simulink model "CardiacDigitalTwin_v2"  (R2026a)
settings: Solver=ode45  StopTime=3600  MaxStep=10
values from neighbouring files (symbols this model uses):
  baroreflex_gain = 0.30    (= 0.3)    [cardiac_params_v2.m]
  baroreflex_tau = 60    [cardiac_params_v2.m]
  baseline_heart_rate = 75    [cardiac_params.m]
  beta_blocker_dose_mg = 60    [cardiac_params.m]
  ec50_mg = 35    [cardiac_params_v2.m]
  emax_bpm = 18    [cardiac_params_v2.m]
  hill_n = 1.5    [cardiac_params_v2.m]
  map_setpoint_mmHg = 94    [cardiac_params_v2.m]
  pk_time_constant = 1800    [cardiac_params.m]
  stroke_volume_mL = 70    [cardiac_params.m]
  svr_mmHg_min_per_L = 18    [cardiac_params.m]
settings Model: Creator=tauilsamuel  LastModifiedBy=tauilsamuel

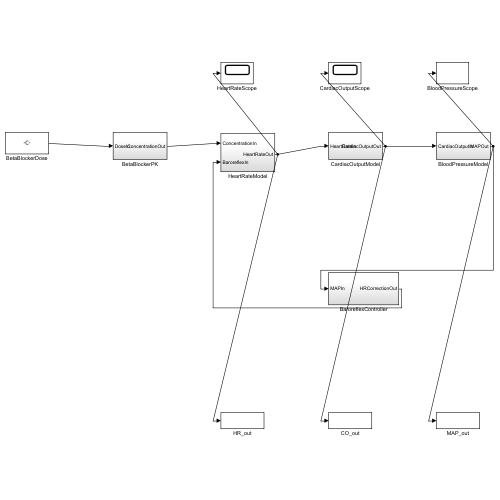
[thumbnail: Simulink's stored preview of the top-level diagram]
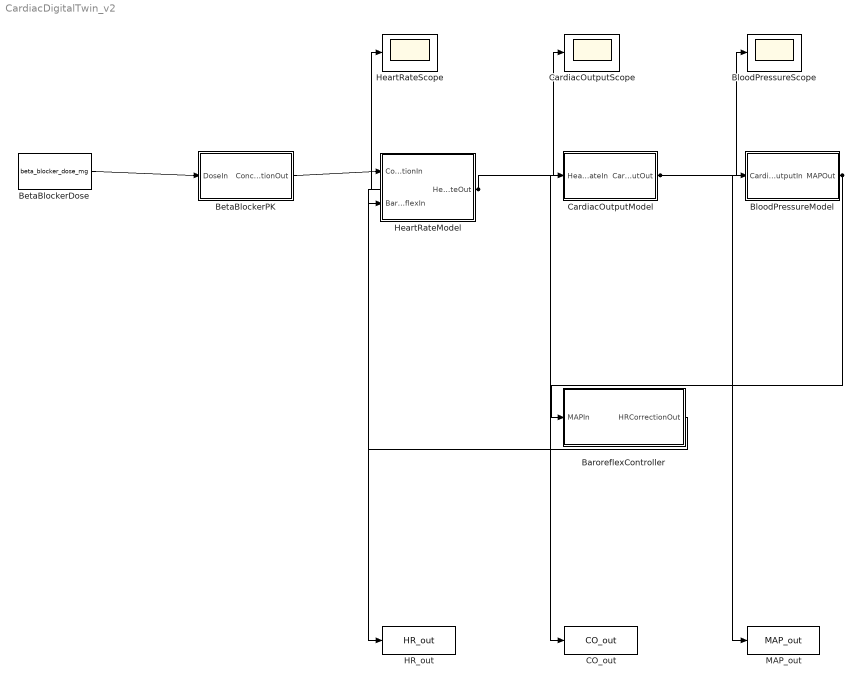
== system CardiacDigitalTwin_v2 ==
  BaroreflexController : Subsystem
  BetaBlockerDose : Constant  Value=beta_blocker_dose_mg
  BetaBlockerPK : Subsystem
  BloodPressureModel : Subsystem
  BloodPressureScope : Scope
  CO_out : ToWorkspace  VariableName=CO_out  SampleTime=-1
  CardiacOutputModel : Subsystem
  CardiacOutputScope : Scope
  HR_out : ToWorkspace  VariableName=HR_out  SampleTime=-1
  HeartRateModel : Subsystem
  HeartRateScope : Scope
  MAP_out : ToWorkspace  VariableName=MAP_out  SampleTime=-1
  wires:
  BetaBlockerDose/1 -> BetaBlockerPK/1(DoseIn)
  BetaBlockerPK/1(ConcentrationOut) -> HeartRateModel/1(ConcentrationIn)
  HeartRateModel/1(HeartRateOut) -> CardiacOutputModel/1(HeartRateIn), HeartRateScope/1, HR_out/1
  CardiacOutputModel/1(CardiacOutputOut) -> BloodPressureModel/1(CardiacOutputIn), CardiacOutputScope/1, CO_out/1
  BloodPressureModel/1(MAPOut) -> BaroreflexController/1(MAPIn), BloodPressureScope/1, MAP_out/1
  BaroreflexController/1(HRCorrectionOut) -> HeartRateModel/2(BaroreflexIn)

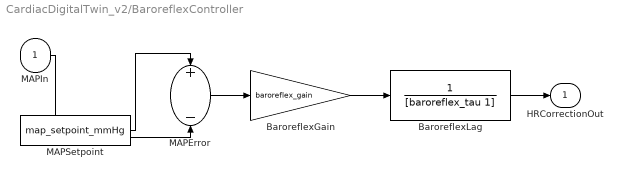
== system CardiacDigitalTwin_v2/BaroreflexController ==
  MAPIn : Inport
  BaroreflexGain : Gain  Gain=baroreflex_gain
  BaroreflexLag : TransferFcn  Denominator=[baroreflex_tau 1]
  MAPError : Sum  Inputs=+-
  MAPSetpoint : Constant  Value=map_setpoint_mmHg
  HRCorrectionOut : Outport
  wires:
  MAPSetpoint/1 -> MAPError/1
  MAPIn/1 -> MAPError/2
  MAPError/1 -> BaroreflexGain/1
  BaroreflexGain/1 -> BaroreflexLag/1
  BaroreflexLag/1 -> HRCorrectionOut/1

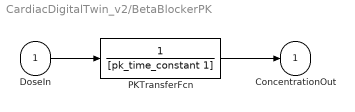
== system CardiacDigitalTwin_v2/BetaBlockerPK ==
  DoseIn : Inport
  PKTransferFcn : TransferFcn  Denominator=[pk_time_constant 1]
  ConcentrationOut : Outport
  wires:
  DoseIn/1 -> PKTransferFcn/1
  PKTransferFcn/1 -> ConcentrationOut/1

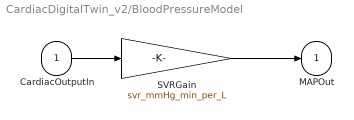
== system CardiacDigitalTwin_v2/BloodPressureModel ==
  CardiacOutputIn : Inport
  SVRGain : Gain  Gain=svr_mmHg_min_per_L
  MAPOut : Outport
  wires:
  CardiacOutputIn/1 -> SVRGain/1
  SVRGain/1 -> MAPOut/1

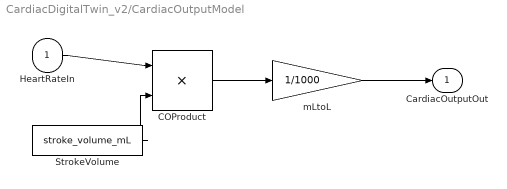
== system CardiacDigitalTwin_v2/CardiacOutputModel ==
  HeartRateIn : Inport
  COProduct : Product  Inputs=**
  StrokeVolume : Constant  Value=stroke_volume_mL
  mLtoL : Gain  Gain=1/1000
  CardiacOutputOut : Outport
  wires:
  HeartRateIn/1 -> COProduct/1
  StrokeVolume/1 -> COProduct/2
  COProduct/1 -> mLtoL/1
  mLtoL/1 -> CardiacOutputOut/1

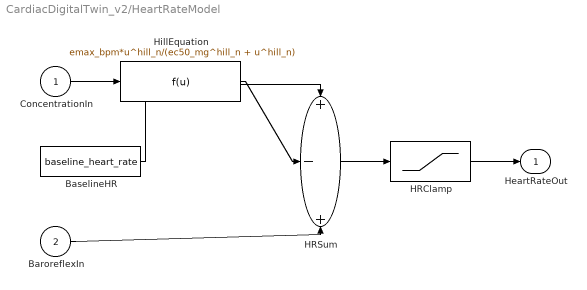
== system CardiacDigitalTwin_v2/HeartRateModel ==
  ConcentrationIn : Inport
  BaroreflexIn : Inport  Port=2
  BaselineHR : Constant  Value=baseline_heart_rate
  HRClamp : Saturate  UpperLimit=180  LowerLimit=40
  HRSum : Sum  Inputs=+-+
  HillEquation : Fcn  Expr=emax_bpm*u^hill_n/(ec50_mg^hill_n + u^hill_n)
  HeartRateOut : Outport
  wires:
  ConcentrationIn/1 -> HillEquation/1
  BaselineHR/1 -> HRSum/1
  HillEquation/1 -> HRSum/2
  BaroreflexIn/1 -> HRSum/3
  HRSum/1 -> HRClamp/1
  HRClamp/1 -> HeartRateOut/1
